simulink model "parameter_optimization_model"  (R2020b)
settings: Solver=VariableStepAuto  StartTime=0.0  StopTime=t_end  RelTol=1e-3
undefined symbols (not defined in the file): curve, Cvi, lambda, MRO2, Pai, Q, tau_a, tau_v, Vl, Vt
settings Model: Creator=Sam  LastModifiedBy=Sam

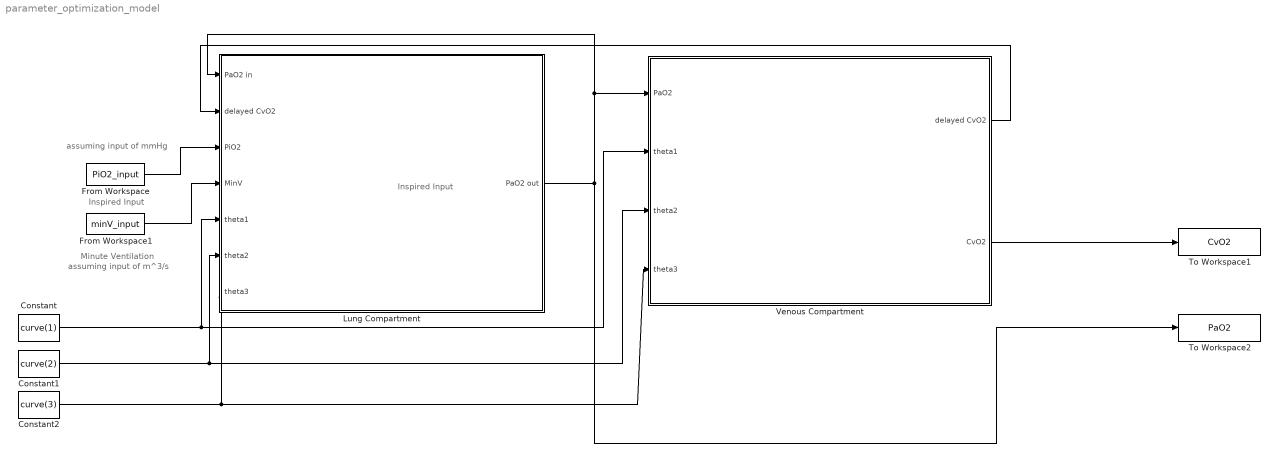
== system parameter_optimization_model ==
  note: Minute Ventilation
  note: Inspired Input
  note: Inspired Input
  note: assuming input of mmHg
  note: assuming input of m^3/s
  Constant : Constant  Value=curve(1)
  Constant1 : Constant  Value=curve(2)
  Constant2 : Constant  Value=curve(3)
  From Workspace : FromWorkspace  VariableName=PiO2_input
  From Workspace1 : FromWorkspace  VariableName=minV_input
  Lung Compartment : Subsystem
  To Workspace1 : ToWorkspace  VariableName=CvO2  SaveFormat=Timeseries  SampleTime=-1
  To Workspace2 : ToWorkspace  VariableName=PaO2  SaveFormat=Timeseries  SampleTime=-1
  Venous Compartment : Subsystem
  wires:
  Venous Compartment/1(delayed CvO2) -> Lung Compartment/2(delayed CvO2)
  Lung Compartment/1(PaO2 out) -> Lung Compartment/1(PaO2 in), Venous Compartment/1(PaO2), To Workspace2/1
  From Workspace/1 -> Lung Compartment/3(PiO2)
  Venous Compartment/2(CvO2) -> To Workspace1/1
  Constant/1 -> Venous Compartment/2(theta1), Lung Compartment/5(theta1)
  Constant1/1 -> Venous Compartment/3(theta2), Lung Compartment/6(theta2)
  Constant2/1 -> Lung Compartment/7(theta3), Venous Compartment/4(theta3)
  From Workspace1/1 -> Lung Compartment/4(MinV)

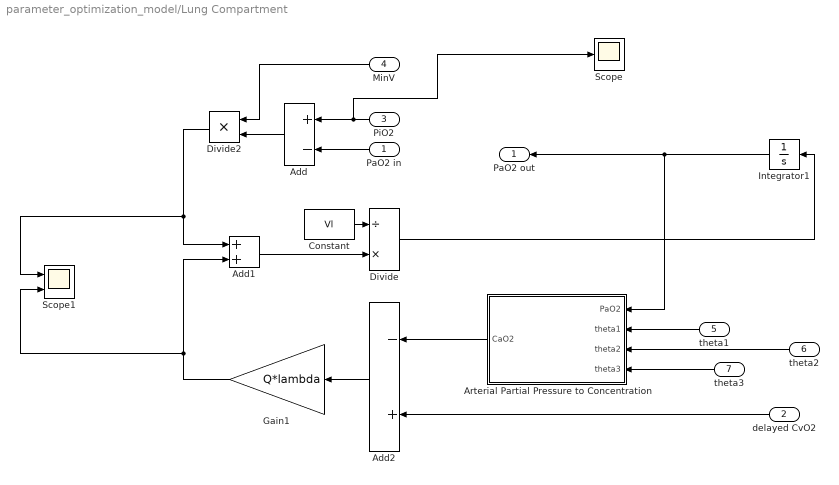
== system parameter_optimization_model/Lung Compartment ==
  PaO2 in : Inport
  delayed CvO2 : Inport  Port=2
  PiO2 : Inport  Port=3
  MinV : Inport  Port=4
  theta1 : Inport  Port=5
  theta2 : Inport  Port=6
  theta3 : Inport  Port=7
  Add : Sum  Inputs=+-
  Add1 : Sum
  Add2 : Sum  Inputs=-+
  Arterial Partial Pressure to Concentration : MATLAB Function  TreatAsAtomicUnit=on
  Constant : Constant  Value=Vl
  Divide : Product  Inputs=/*
  Divide2 : Product  Inputs=**
  Gain1 : Gain  Gain=Q*lambda
  Integrator1 : Integrator  InitialCondition=Pai
  Scope : Scope
  Scope1 : Scope  NumInputPorts=2
  PaO2 out : Outport
  wires:
  Divide/1 -> Integrator1/1
  Add1/1 -> Divide/2
  Constant/1 -> Divide/1
  Add/1 -> Divide2/2
  Add2/1 -> Gain1/1
  PaO2 in/1 -> Add/2
  MinV/1 -> Divide2/1
  Divide2/1 -> Scope1/1, Add1/1
  Gain1/1 -> Scope1/2, Add1/2
  Integrator1/1 -> Arterial Partial Pressure to Concentration/1(PaO2), PaO2 out/1
  PiO2/1 -> Scope/1, Add/1
  delayed CvO2/1 -> Add2/2
  Arterial Partial Pressure to Concentration/1(CaO2) -> Add2/1
  theta1/1 -> Arterial Partial Pressure to Concentration/2(theta1)
  theta2/1 -> Arterial Partial Pressure to Concentration/3(theta2)
  theta3/1 -> Arterial Partial Pressure to Concentration/4(theta3)

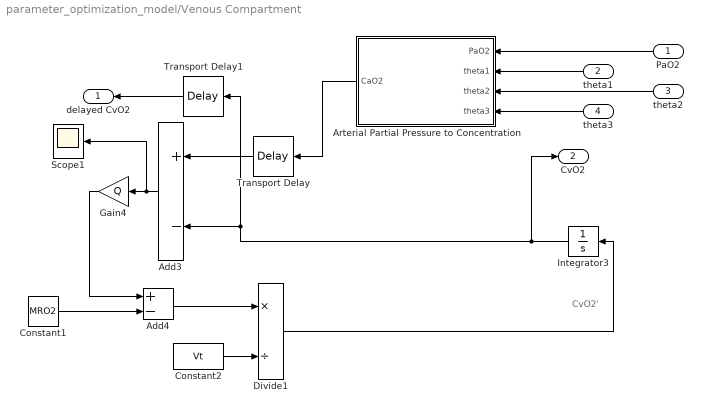
== system parameter_optimization_model/Venous Compartment ==
  note: CvO2'
  PaO2 : Inport
  theta1 : Inport  Port=2
  theta2 : Inport  Port=3
  theta3 : Inport  Port=4
  Add3 : Sum  Inputs=+-
  Add4 : Sum  Inputs=+-
  Arterial Partial Pressure to Concentration : MATLAB Function  TreatAsAtomicUnit=on
  Constant1 : Constant  Value=MRO2
  Constant2 : Constant  Value=Vt
  Divide1 : Product  Inputs=*/
  Gain4 : Gain  Gain=Q
  Integrator3 : Integrator  InitialCondition=Cvi
  Scope1 : Scope
  Transport Delay : TransportDelay  DelayTime=tau_a
  Transport Delay1 : TransportDelay  DelayTime=tau_v
  delayed CvO2 : Outport
  CvO2 : Outport  Port=2
  wires:
  Transport Delay1/1 -> delayed CvO2/1
  Constant1/1 -> Add4/2
  Transport Delay/1 -> Add3/1
  Gain4/1 -> Add4/1
  Add3/1 -> Scope1/1, Gain4/1
  Divide1/1 -> Integrator3/1
  Arterial Partial Pressure to Concentration/1(CaO2) -> Transport Delay/1
  Integrator3/1 -> Transport Delay1/1, Add3/2, CvO2/1
  Constant2/1 -> Divide1/2
  Add4/1 -> Divide1/1
  theta1/1 -> Arterial Partial Pressure to Concentration/2(theta1)
  theta3/1 -> Arterial Partial Pressure to Concentration/4(theta3)
  theta2/1 -> Arterial Partial Pressure to Concentration/3(theta2)
  PaO2/1 -> Arterial Partial Pressure to Concentration/1(PaO2)

== matlab function parameter_optimization_model/Lung Compartment/Arterial Partial Pressure to Concentration ==
  data: PaO2 input; CaO2 output; theta1 input; theta2 input; theta3 input
function CaO2 = O2_dissociation(PaO2, theta1, theta2, theta3)
CaO2 = dissociation_curve(PaO2, theta1, theta2, theta3);
% SaO2 = theta3*(PaO2.^3 + theta1*PaO2)./...
%         (PaO2.^3 + theta1*PaO2 + theta2);
% CaO2 = (1.34*16*SaO2 + 0.0031*PaO2)/100;

== matlab function parameter_optimization_model/Venous Compartment/Arterial Partial Pressure to Concentration ==
  data: PaO2 input; CaO2 output; theta1 input; theta2 input; theta3 input
function CaO2 = O2_dissociation(PaO2, theta1, theta2, theta3)
% CaO2 = dissociation_curve(PaO2, theta1, theta2, theta3);
SaO2 = theta3*(PaO2.^3 + theta1*PaO2)./...
        (PaO2.^3 + theta1*PaO2 + theta2);
CaO2 = (1.34*16*SaO2 + 0.0031*PaO2)/100;
